simulink model "LIN_Corner"  (R2016b)
settings: Solver=FixedStepAuto  StartTime=0.0  StopTime=3  FixedStep=0.001  RelTol=1e-3
values from neighbouring files (symbols this model uses):
  A = [zeros(3,3), dPhiMat, zeros(3,3) ... (first row only)    [ParameterInit.m]    (also in SimulinkInit.m = SSc.A; controller_design_lqr.m = SSd.A)
  B = [zeros(3,3); -I_K_inv; I_R_inv]    [ParameterInit.m]    (also in SimulinkInit.m = SSc.B; controller_design_lqr.m = SSd.B)
  Kd = K_unlimited    [LinearSimulationScript.m]    (also in controller_design_lqr.m = KKd * [eye(7), zeros(7,2)]/T_K)
  x0 = [0; 0.11; 0.08; 0; 1; -2; 3; -16; 0]    [LinearSimulationScript.m]    (also in SimulinkInit.m = [0; 0.5; 0.2; 0; 2; -1; 1; 0; 0])
  x_offset = [0; 0.02; 0.0; 0; 0; 0; 0; 0; 0]    [SimulinkInit.m]
settings Model: Creator=michael  LastModifiedBy=ich

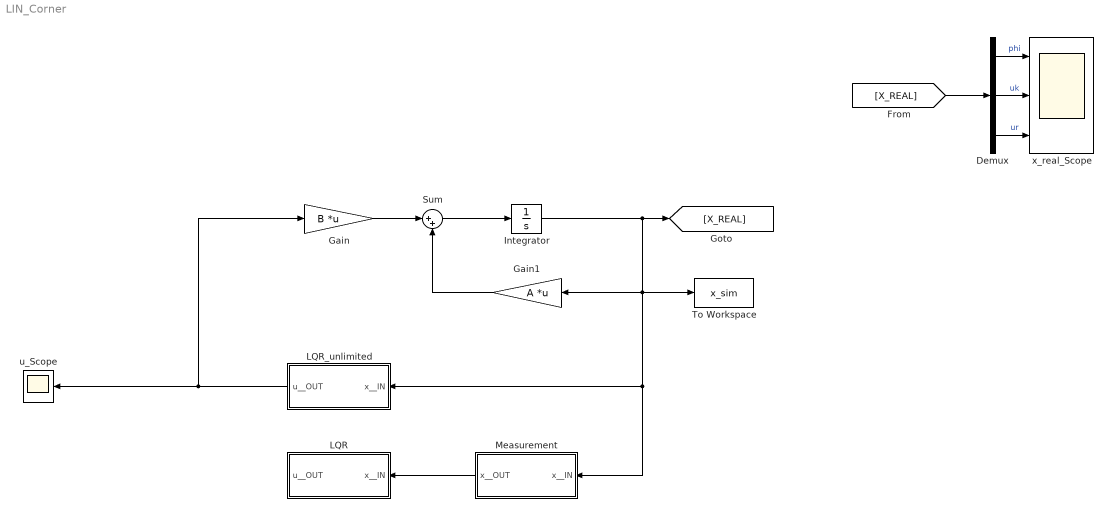
== system LIN_Corner ==
  Demux : Demux  Outputs=3
  Gain : Gain  Gain=B  Multiplication=Matrix(K*u) (u vector)
  Gain1 : Gain  Gain=A  Multiplication=Matrix(K*u) (u vector)
  Integrator : Integrator  InitialCondition=x0
  LQR : Subsystem
  LQR_unlimited : Subsystem
  Measurement : Subsystem
  Sum : Sum  Inputs=|++
  To Workspace : ToWorkspace  VariableName=x_sim  SaveFormat=Structure With Time  SampleTime=-1
  u_Scope : Scope
  x_real_Scope : Scope  NumInputPorts=3
  wires:
  Gain/1 -> Sum/1
  Sum/1 -> Integrator/1
  Gain1/1 -> Sum/2
  Integrator/1 -> [X_REAL], Gain1/1, To Workspace/1, LQR_unlimited/1(x__IN), Measurement/1(x__IN)
  [X_REAL] -> Demux/1
  Demux/1 -> x_real_Scope/1  "phi"
  Demux/2 -> x_real_Scope/2  "uk"
  Demux/3 -> x_real_Scope/3  "ur"
  Measurement/1(x__OUT) -> LQR/1(x__IN)
  LQR_unlimited/1(u__OUT) -> Gain/1, u_Scope/1

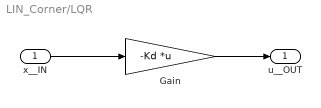
== system LIN_Corner/LQR ==
  x__IN : Inport  SampleTime=0.02
  Gain : Gain  Gain=-Kd  Multiplication=Matrix(K*u) (u vector)
  u__OUT : Outport
  wires:
  x__IN/1 -> Gain/1
  Gain/1 -> u__OUT/1

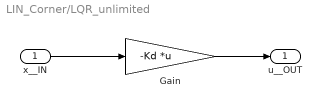
== system LIN_Corner/LQR_unlimited ==
  x__IN : Inport  SampleTime=0.02
  Gain : Gain  Gain=-Kd  Multiplication=Matrix(K*u) (u vector)
  u__OUT : Outport
  wires:
  Gain/1 -> u__OUT/1
  x__IN/1 -> Gain/1

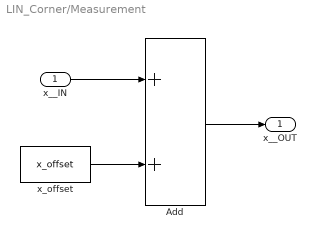
== system LIN_Corner/Measurement ==
  x__IN : Inport  SampleTime=0.02
  Add : Sum
  x_offset : Constant  Value=x_offset
  x__OUT : Outport
  wires:
  Add/1 -> x__OUT/1
  x__IN/1 -> Add/1
  x_offset/1 -> Add/2
